simulink model "test2_model"  (R2021b)
settings: Solver=ode23tb  StartTime=0.0  StopTime=ctrl_tm  RelTol=1e-3
values from neighbouring files (symbols this model uses):
  A = J    (= 0.066829)    [test_big.m]    (also in test_small.m = 0.000254045)
  B = b_m + b + (b/(N^2*n_g))    (= 0.00010739)    [test_big.m]    (also in test_small.m = 6e-07)
  ctrl_k = k    (= 0)    [controller_init.m]    (also in controller_init2.m = 1; controller_init3.m = 1)
  ctrl_len = len    (= 30)    [controller_init.m]    (also in controller_init2.m; controller_init3.m = 200)
  ctrl_tm = tm    (= 7.5)    [controller_init.m]    (also in controller_init2.m = 3; controller_init3.m = 20)
  D = (mu_s*cos(angl) + sin(angl)) * r_p*(m_l+m_b)*g/(N*n_g)    [test_big.m]    (also in test_small.m = 0.113379075)
  Ke = 0.0537    [test_big.m]    (also in test_small.m = 0.0168)
  L = 0.0308e-3    (= 3.08e-05)    [test_big.m]    (also in test_small.m = 0.000333)
  MP_ON = 1    [test_big.m]
  N = (1:0.1:50)    [gear_ratio_code_1.m]    (also in test_big.m = 1; test_small.m = 1)
  R = 0.0821    [test_big.m]    (also in test_small.m = 3.17)
  r_p = 0.5e-1    (= 0.05)    [test_big.m]    (also in test_small.m = 0.005)
  V = 24    [test_big.m]    (also in test_small.m = 12)
libraries: slpidlib x1, simulink x1, RCTblocks x1, eePwmGenerator x1
settings Model: Creator=marcelafunyah  LastModifiedBy=marcelafunyah

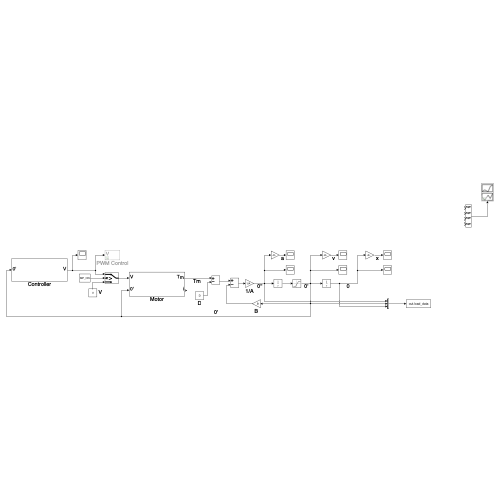
[thumbnail: Simulink's stored preview of the top-level diagram]
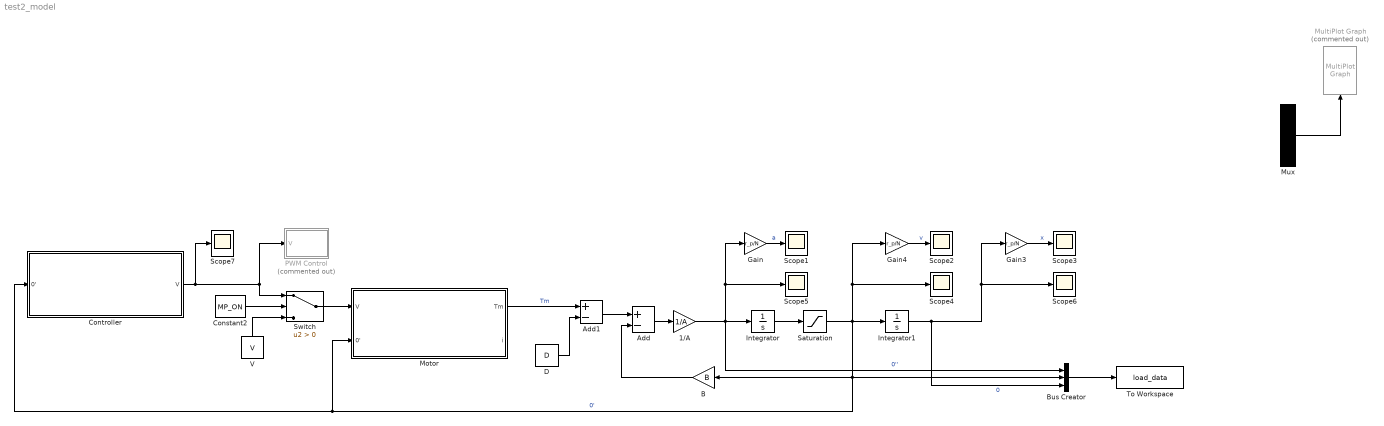
== system test2_model ==
  1/A : Gain  Gain=1/A
  Add : Sum  Inputs=+-
  Add1 : Sum  Inputs=+-
  B : Gain  Gain=B
  Bus Creator : BusCreator  Inputs=3
  Constant2 : Constant  Value=MP_ON
  Controller : Subsystem
  D : Constant  Value=D
  Gain : Gain  Gain=r_p/N
  Gain3 : Gain  Gain=r_p/N
  Gain4 : Gain  Gain=r_p/N
  Integrator : Integrator
  Integrator1 : Integrator
  Motor : Subsystem
  MultiPlot Graph : RCTblocks/MultiPlot Graph  Tag=MultiPlot  Commented=on  tmin=0  tmax=30  ymin=-inf  ymax=inf  Tsamp=-1  vnamesave=multisimout
      settings: SourceProductBaseCode=RC
  Mux : Mux
      settings: DisplayOption=signals
  PWM Control : Subsystem  Commented=on
  Saturation : Saturate  UpperLimit=inf  LowerLimit=0
  Scope{1..7} (7 alike) : Scope
  Switch : Switch  Criteria=u2 > Threshold
  To Workspace : ToWorkspace  VariableName=load_data  SaveFormat=Timeseries  SampleTime=-1
  V : Constant  Value=V
  wires:
  Integrator/1 -> Saturation/1
  Integrator1/1 -> Bus Creator/3, Gain3/1, Scope6/1  "0"
  1/A/1 -> Bus Creator/1, Gain/1, Scope5/1, Integrator/1  "0''"
  B/1 -> Add/2
  Gain/1 -> Scope1/1  "a"
  Gain4/1 -> Scope2/1  "v"
  Gain3/1 -> Scope3/1  "x"
  Add/1 -> 1/A/1
  D/1 -> Add1/2
  Add1/1 -> Add/1
  Motor/1(Tm) -> Add1/1  "Tm"
  Mux/1 -> MultiPlot Graph/1
  Controller/1(V) -> Scope7/1, PWM Control/1(V), Switch/1
  V/1 -> Switch/3
  Saturation/1 -> Gain4/1, Scope4/1, Controller/1(0'), Motor/2(0'), Bus Creator/2, B/1, Integrator1/1  "0'"
  Switch/1 -> Motor/1(V)
  Constant2/1 -> Switch/2
  Bus Creator/1 -> To Workspace/1

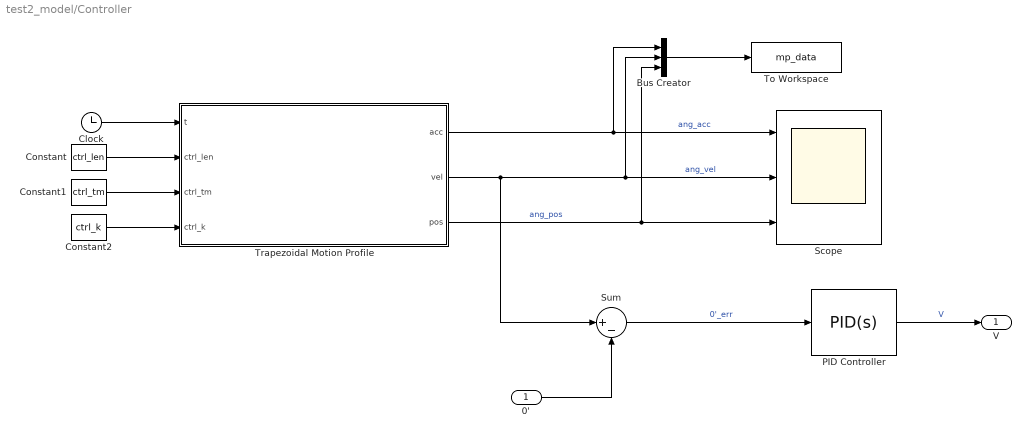
== system test2_model/Controller ==
  0' : Inport
  Bus Creator : BusCreator  Inputs=3
  Clock : Clock
  Constant : Constant  Value=ctrl_len
  Constant1 : Constant  Value=ctrl_tm
  Constant2 : Constant  Value=ctrl_k
  PID Controller : slpidlib/PID Controller  Controller=PID  Form=Parallel  TimeDomain=Continuous-time  UseExternalTs=off  SampleTime=-1  IntegratorMethod=Forward Euler  FilterMethod=Forward Euler  ControllerParametersSource=internal  P=1061.95540542735  I=473914.78302098  D=0.419694726373319  UseFilter=on  N=693808.007297607  TunerSelectOption=Transfer Function Based (PID Tuner App)  InitialConditionSource=internal  InitialConditionForIntegrator=0  InitialConditionForFilter=0  DifferentiatorICPrevScaledInput=0  ExternalReset=none  TrackingMode=off  Kt=1  LimitOutput=on  SatLimitsSource=internal  UpperSaturationLimit=12  LowerSaturationLimit=0  LinearizeAsGain=on  AntiWindupMode=none  Kb=1  POutMin=[]  POutMax=[]  IOutMin=[]  IOutMax=[]  DOutMin=[]  DOutMax=[]  NOutMin=[]  NOutMax=[]  SumOutMin=[]  SumOutMax=[]  SaturationOutMin=[]  SaturationOutMax=[]  PParamMin=[]  PParamMax=[]  IParamMin=[]  IParamMax=[]  DParamMin=[]  DParamMax=[]  NParamMin=[]  NParamMax=[]  KbParamMin=[]  KbParamMax=[]  KtParamMin=[]  KtParamMax=[]  KbOutMin=[]  KbOutMax=[]  KtOutMin=[]  KtOutMax=[]  IntegratorOutMin=[]  IntegratorOutMax=[]  FilterOutMin=[]  FilterOutMax=[]  SumI1OutMin=[]  SumI1OutMax=[]  SumI2OutMin=[]  SumI2OutMax=[]  SumI3OutMin=[]  SumI3OutMax=[]  SumI4OutMin=[]  SumI4OutMax=[]  SumDOutMin=[]  SumDOutMax=[]  DifferentiatorOutMin=[]  DifferentiatorOutMax=[]  FilterDiffOutCoefMin=[]  FilterDiffOutCoefMax=[]  ReciprocalOutMin=[]  ReciprocalOutMax=[]  SumDenOutMin=[]  SumDenOutMax=[]  SumNumOutMin=[]  SumNumOutMax=[]  DivideOutMin=[]  DivideOutMax=[]  UdiffTsProdOutMin=[]  UdiffTsProdOutMax=[]  NTsProdOutMin=[]  NTsProdOutMax=[]  UintegralTsProdOutMin=[]  UintegralTsProdOutMax=[]  UngainTsProdOutMin=[]  UngainTsProdOutMax=[]  IntegratorContinuousStateAttributes=''  IntegratorStateMustResolveToSignalObject=off  IntegratorRTWStateStorageClass=Auto  FilterContinuousStateAttributes=''  FilterStateMustResolveToSignalObject=off  FilterRTWStateStorageClass=Auto  ParallelPVariant=InternalParameters  IdealPVariant=Disabled  IVariant=InternalParameters  DVariant=InternalParameters  IntegratorVariant=Continuous  SatVariant=Enabled  AWVariant=Passthrough  PCopyVariant=Disabled  TRVariant=Disabled  FdbkBlocksVariant=Forward  IdealPFdbkVariant=Disabled  SatFdbkVariant=Disabled  DerivativeFilterVariant=ContFilter  NVariant=InternalParameters  NCopyVariant=Disabled  FilterICVariant=InternalICsFilter  IntegratorICVariant=InternalICs  ExternalResetVariant=Disabled  TRSumVariant=Passthrough  SumFdbkVariant=Disabled  SumVariant=Sum_PID  TsampFilterVariant=InternalTs  TsampNgainVariant=Passthrough  TsampIntegralVariant=Passthrough  ExternalSaturationOutDataTypeStr=Inherit: Same as second input
  Scope : Scope  NumInputPorts=3
  Sum : Sum  Inputs=|+-
  To Workspace : ToWorkspace  VariableName=mp_data  SaveFormat=Timeseries  SampleTime=-1
      settings: Save2DSignal=2-D array (concatenate along first dimension)
  Trapezoidal Motion Profile : MATLAB Function  TreatAsAtomicUnit=on
  V : Outport
  wires:
  Trapezoidal Motion Profile/3(pos) -> Bus Creator/3, Scope/3  "ang_pos"
  Trapezoidal Motion Profile/1(acc) -> Bus Creator/1, Scope/1  "ang_acc"
  Trapezoidal Motion Profile/2(vel) -> Bus Creator/2, Scope/2, Sum/1  "ang_vel"
  Clock/1 -> Trapezoidal Motion Profile/1(t)
  Sum/1 -> PID Controller/1  "0'_err"
  PID Controller/1 -> V/1  "V"
  0'/1 -> Sum/2
  Constant/1 -> Trapezoidal Motion Profile/2(ctrl_len)
  Constant1/1 -> Trapezoidal Motion Profile/3(ctrl_tm)
  Constant2/1 -> Trapezoidal Motion Profile/4(ctrl_k)
  Bus Creator/1 -> To Workspace/1

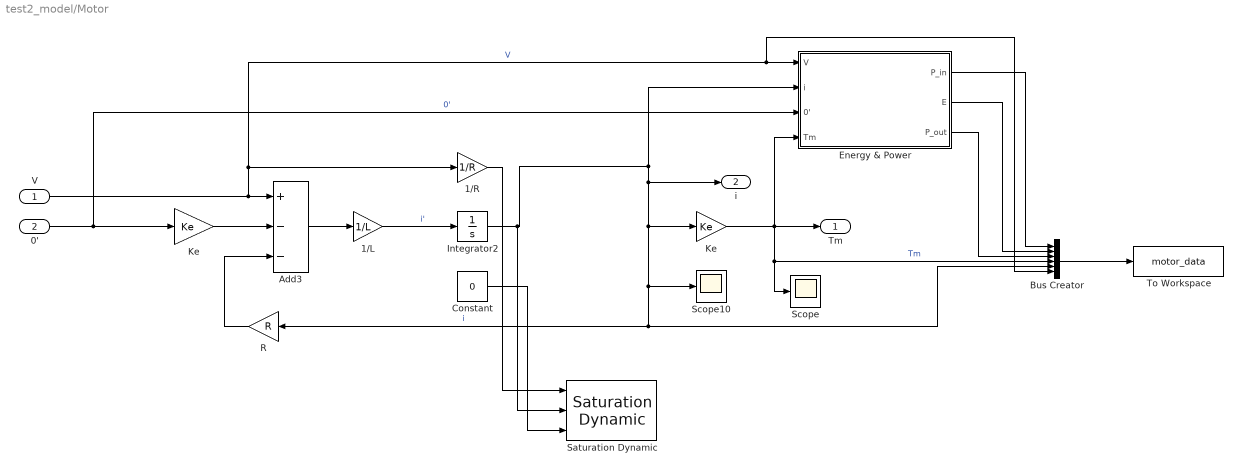
== system test2_model/Motor ==
  V : Inport
  0' : Inport  Port=2
  1/L : Gain  Gain=1/L
  1/R : Gain  Gain=1/R
  Add3 : Sum  Inputs=+--
  Bus Creator : BusCreator  Inputs=6
  Constant : Constant  Value=0
  Energy & Power : Subsystem
  Integrator2 : Integrator
  Ke : Gain  Gain=Ke
  "Ke " : Gain  Gain=Ke
  R : Gain  Gain=R
  Saturation Dynamic : simulink/Discontinuities/Saturation Dynamic  OutMin=[]  OutMax=[]  OutDataTypeStr=Inherit: Same as second input  OutDataType=fixdt(1, 16)  OutScaling=2^-10  DoSatur=off
  Scope : Scope
  Scope10 : Scope
  To Workspace : ToWorkspace  VariableName=motor_data  SaveFormat=Timeseries  SampleTime=-1
  Tm : Outport
  i : Outport  Port=2
  wires:
  R/1 -> Add3/3
  Add3/1 -> 1/L/1
  "Ke "/1 -> Energy & Power/4(Tm), Scope/1, Bus Creator/4, Tm/1  "Tm"
  1/L/1 -> Integrator2/1  "i'"
  Ke/1 -> Add3/2
  V/1 -> Bus Creator/6, Energy & Power/1(V), 1/R/1, Add3/1  "V"
  0'/1 -> Ke/1, Energy & Power/3(0')  "0'"
  Integrator2/1 -> Bus Creator/5, R/1, Scope10/1, "Ke "/1, i/1, Energy & Power/2(i), Saturation Dynamic/2  "i"
  1/R/1 -> Saturation Dynamic/1
  Constant/1 -> Saturation Dynamic/3
  Bus Creator/1 -> To Workspace/1
  Energy & Power/3(P_out) -> Bus Creator/3
  Energy & Power/2(E) -> Bus Creator/2
  Energy & Power/1(P_in) -> Bus Creator/1

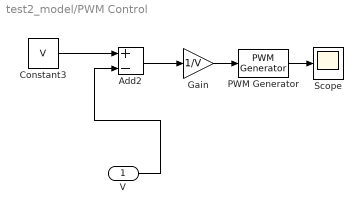
== system test2_model/PWM Control ==
  V : Inport
  Add2 : Sum  Inputs=+-
  Constant3 : Constant  Value=V
  Gain : Gain  Gain=1/V
  PWM Generator : eePwmGenerator/PWM Generator  CarrCount=Up  Tper=0.001  Tdelay=0  Ts=0
  Scope : Scope
  wires:
  PWM Generator/1 -> Scope/1
  Gain/1 -> PWM Generator/1
  Constant3/1 -> Add2/1
  V/1 -> Add2/2
  Add2/1 -> Gain/1

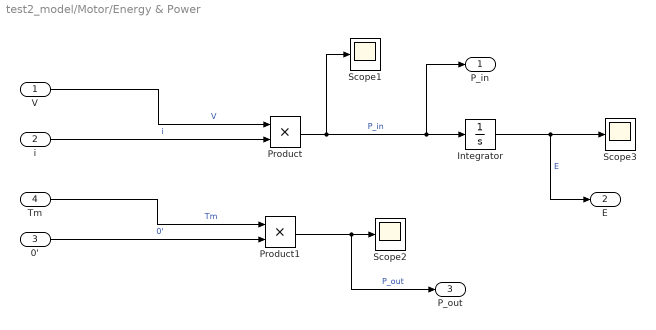
== system test2_model/Motor/Energy & Power ==
  V : Inport
  i : Inport  Port=2
  0' : Inport  Port=3
  Tm : Inport  Port=4
  Integrator : Integrator
  Product : Product
  Product1 : Product
  Scope1 : Scope
  Scope2 : Scope
  Scope3 : Scope
  P_in : Outport
  E : Outport  Port=2
  P_out : Outport  Port=3
  wires:
  V/1 -> Product/1  "V"
  i/1 -> Product/2  "i"
  Product/1 -> P_in/1, Integrator/1, Scope1/1  "P_in"
  Integrator/1 -> E/1, Scope3/1  "E"
  Tm/1 -> Product1/1  "Tm"
  0'/1 -> Product1/2  "0'"
  Product1/1 -> P_out/1, Scope2/1  "P_out"

== matlab function test2_model/Controller/Trapezoidal Motion Profile ==
  data: t input; acc output; vel output; pos output; ctrl_len input; ctrl_tm input; ctrl_k input
function [acc,vel,pos] = fcn(t, ctrl_len, ctrl_tm, ctrl_k)

%     len = 16*pi;
%     tm = 7;
%     
%     
%     % max_ang_acc = 0.01;
%     % k = sqrt(1 - (4*len/tm^2 * max_ang_acc));
%     
%     k = 0.5;


    len = ctrl_len;
    tm = ctrl_tm;
    k = ctrl_k;

    
%     max_ang_vel = (2/(1+k)) * (len/tm);
    % max_ang_vel = 0; k = (2*L/(tm*max_ang_vel)) - 1;
    
%     ta = 0;
%     tb = ta + 0.5 * (tm - k*tm);
%     tc = tb + k*tm;
%     td = tm;
%     
%     alpha = (4/(1-k^2)) * (len/tm^2);
%     
%     if (t>=ta) && (t<=tb)
%         ang_acc = alpha;
%         ang_vel = alpha * t;
%         ang_pos = 0.5 * alpha * t^2; 
%     elseif (t>tb) && (t<=tc)
%         ang_acc = 0;
%         ang_vel = alpha * tb;
%         ang_pos = (0.5 * alpha * tb^2) + (alpha * tb) * (t - tb); 
%     elseif (t>tc) && (t<=td)
%         ang_acc = -alpha;
%         ang_vel = (alpha * tb) - alpha*(t-tc);
%         ang_pos = (0.5 * alpha * tb^2) + (alpha * tb) * (tc - tb) + (alpha * tb) * (t - tc) + (alpha * tc) * (t - tc) - 0.5 * alpha * (t^2 - tc^2);
%     else
%         ang_acc = 0;
%         ang_vel = 0;
%         ang_pos = (0.5 * alpha * tb^2) + (alpha * tb) * (tc - tb) + (alpha * tb) * (tm - tc) + (alpha * tc) * (tm - tc) - 0.5 * alpha * (tm^2 - tc^2);
%     end
    

    t0 = 0;
    ta = t0 + 0.5 * (tm - k*tm);
    tb = ta + k*tm;
    td = tm;
    
    alpha = (4/(1-k^2)) * (len/tm^2);
    
    if (t>=t0) && (t<=ta)
        ang_acc = alpha;
        ang_vel = alpha * t;
        ang_pos = 0.5 * alpha * t^2; 
    elseif (t>ta) && (t<=tb)
        ang_acc = 0;
        ang_vel = alpha * ta;
        ang_pos = (0.5 * alpha * ta^2) + (alpha * ta) * (t - ta); 
    elseif (t>tb) && (t<=td)
        ang_acc = -alpha;
        ang_vel = (alpha * ta) - alpha*(t-tb);
        ang_pos = (0.5 * alpha * ta^2) + (alpha * ta) * (tb - ta) + (alpha * ta) * (t - tb) + (alpha * tb) * (t - tb) - 0.5 * alpha * (t^2 - tb^2);
    else
        ang_acc = 0;
        ang_vel = 0;
        ang_pos = (0.5 * alpha * ta^2) + (alpha * ta) * (tb - ta) + (alpha * ta) * (tm - tb) + (alpha * tb) * (tm - tb) - 0.5 * alpha * (tm^2 - tb^2);
    end


acc = ang_acc;
vel = ang_vel;
pos = ang_pos;
